simulink model "huxley_sim"  (R2021b)
settings: Solver=VariableStepAuto  StartTime=0.0  StopTime=2  RelTol=1e-3
values from neighbouring files (symbols this model uses):
  gK = 36    [huxley.m]
  gL = 0.3    [huxley.m]
  gNa = 120    [huxley.m]
  VK = -77    [huxley.m]
  VL = -54.4    [huxley.m]
  VNa = 50    [huxley.m]
  Vrest = -60    [huxley.m]
settings Model: Creator=eraym  LastModifiedBy=eraym

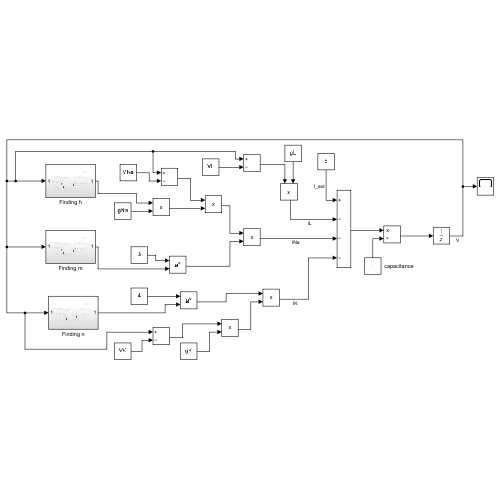
[thumbnail: Simulink's stored preview of the top-level diagram]
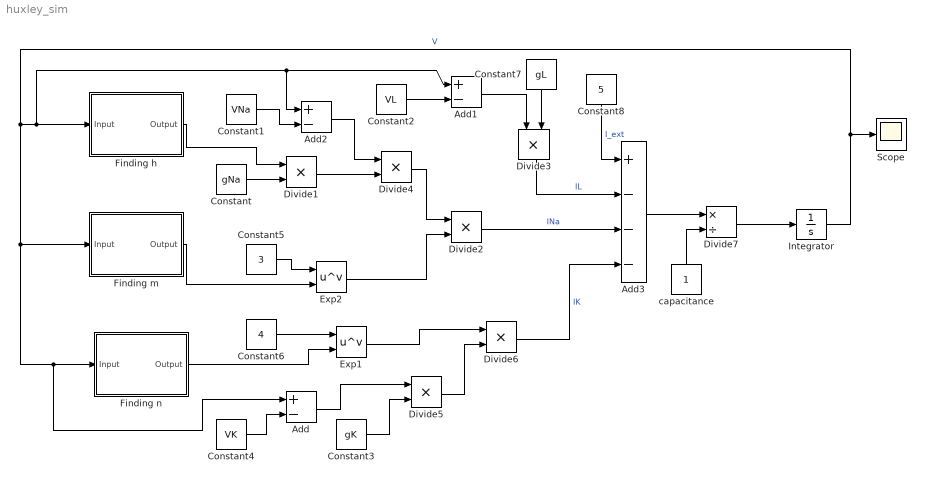
== system huxley_sim ==
  Add : Sum  Inputs=+-
  Add1 : Sum  Inputs=+-
  Add2 : Sum  Inputs=+-
  Add3 : Sum  Inputs=+---
  Constant : Constant  Value=gNa
  Constant1 : Constant  Value=VNa
  Constant2 : Constant  Value=VL
  Constant3 : Constant  Value=gK
  Constant4 : Constant  Value=VK
  Constant5 : Constant  Value=3
  Constant6 : Constant  Value=4
  Constant7 : Constant  Value=gL
  Constant8 : Constant  Value=5
  Divide{1..6} (6 alike) : Product  Inputs=**
  Divide7 : Product  Inputs=*/
  Exp1 : Math  Operator=pow  SaturateOnIntegerOverflow=on
  Exp2 : Math  Operator=pow  SaturateOnIntegerOverflow=on
  Finding h : Subsystem
  Finding m : Subsystem
  Finding n : Subsystem
  Integrator : Integrator
  Scope : Scope
  capacitance : Constant
  wires:
  Finding h/1(Output) -> Divide1/1
  Constant/1 -> Divide1/2
  Divide1/1 -> Divide4/2
  Add2/1 -> Divide4/1
  Constant1/1 -> Add2/2
  Divide4/1 -> Divide2/1
  Finding m/1(Output) -> Exp2/2
  Constant5/1 -> Exp2/1
  Exp2/1 -> Divide2/2
  Divide2/1 -> Add3/3  "INa"
  Divide6/1 -> Add3/4  "IK"
  Finding n/1(Output) -> Exp1/2
  Constant6/1 -> Exp1/1
  Exp1/1 -> Divide6/1
  Divide5/1 -> Divide6/2
  Constant3/1 -> Divide5/2
  Add/1 -> Divide5/1
  Constant4/1 -> Add/2
  Add3/1 -> Divide7/1
  capacitance/1 -> Divide7/2
  Divide7/1 -> Integrator/1
  Integrator/1 -> Scope/1, Add2/1, Add1/1, Finding h/1(Input), Add/1, Finding n/1(Input), Finding m/1(Input)  "V"
  Constant2/1 -> Add1/2
  Add1/1 -> Divide3/1
  Divide3/1 -> Add3/2  "IL"
  Constant7/1 -> Divide3/2
  Constant8/1 -> Add3/1  "I_ext"

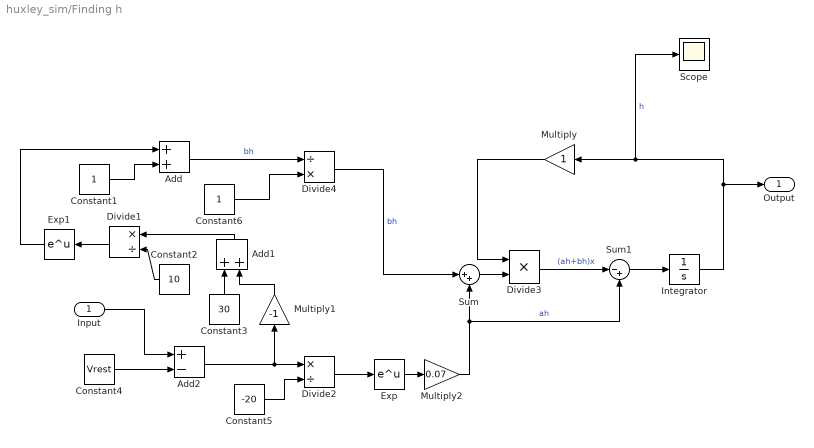
== system huxley_sim/Finding h ==
  Input : Inport
  Add : Sum
  Add1 : Sum
  Add2 : Sum  Inputs=+-
  Constant1 : Constant
  Constant2 : Constant  Value=10
  Constant3 : Constant  Value=30
  Constant4 : Constant  Value=Vrest
  Constant5 : Constant  Value=-20
  Constant6 : Constant
  Divide1 : Product  Inputs=*/
  Divide2 : Product  Inputs=*/
  Divide3 : Product  Inputs=**
  Divide4 : Product  Inputs=/*
  Exp : Math  SaturateOnIntegerOverflow=on
  Exp1 : Math  SaturateOnIntegerOverflow=on
  Integrator : Integrator
  Multiply : Gain
  Multiply1 : Gain  Gain=-1
  Multiply2 : Gain  Gain=0.07
  Scope : Scope
  Sum : Sum  Inputs=|++
  Sum1 : Sum  Inputs=|-+
  Output : Outport
  wires:
  Constant5/1 -> Divide2/2
  Input/1 -> Add2/1
  Sum/1 -> Divide3/2
  Add2/1 -> Divide2/1, Multiply1/1
  Divide1/1 -> Exp1/1
  Constant2/1 -> Divide1/2
  Divide2/1 -> Exp/1
  Exp/1 -> Multiply2/1
  Constant3/1 -> Add1/1
  Constant1/1 -> Add/2
  Add1/1 -> Divide1/1
  Exp1/1 -> Add/1
  Integrator/1 -> Output/1, Multiply/1, Scope/1  "h"
  Constant4/1 -> Add2/2
  Multiply1/1 -> Add1/2
  Multiply2/1 -> Sum1/2, Sum/2  "ah"
  Multiply/1 -> Divide3/1
  Divide4/1 -> Sum/1  "bh"
  Divide3/1 -> Sum1/1  "(ah+bh)x"
  Sum1/1 -> Integrator/1
  Add/1 -> Divide4/1  "bh"
  Constant6/1 -> Divide4/2

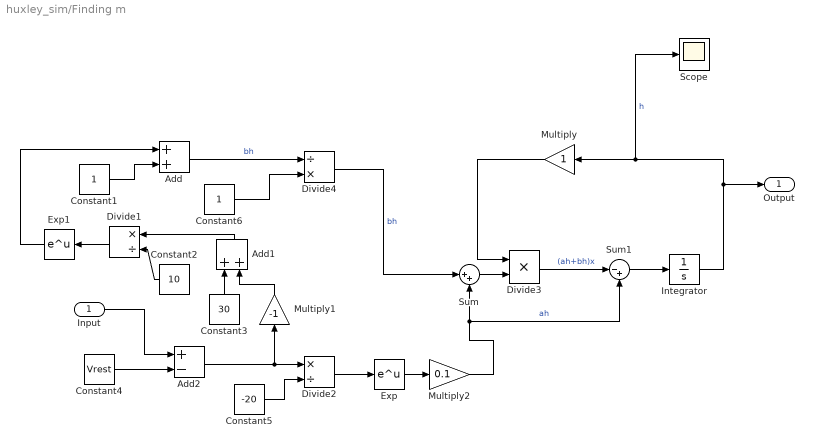
== system huxley_sim/Finding m ==
  Input : Inport
  Add : Sum
  Add1 : Sum
  Add2 : Sum  Inputs=+-
  Constant1 : Constant
  Constant2 : Constant  Value=10
  Constant3 : Constant  Value=30
  Constant4 : Constant  Value=Vrest
  Constant5 : Constant  Value=-20
  Constant6 : Constant
  Divide1 : Product  Inputs=*/
  Divide2 : Product  Inputs=*/
  Divide3 : Product  Inputs=**
  Divide4 : Product  Inputs=/*
  Exp : Math  SaturateOnIntegerOverflow=on
  Exp1 : Math  SaturateOnIntegerOverflow=on
  Integrator : Integrator
  Multiply : Gain
  Multiply1 : Gain  Gain=-1
  Multiply2 : Gain  Gain=0.1
  Scope : Scope
  Sum : Sum  Inputs=|++
  Sum1 : Sum  Inputs=|-+
  Output : Outport
  wires:
  Constant5/1 -> Divide2/2
  Input/1 -> Add2/1
  Sum/1 -> Divide3/2
  Add2/1 -> Divide2/1, Multiply1/1
  Divide1/1 -> Exp1/1
  Constant2/1 -> Divide1/2
  Divide2/1 -> Exp/1
  Exp/1 -> Multiply2/1
  Constant3/1 -> Add1/1
  Constant1/1 -> Add/2
  Add1/1 -> Divide1/1
  Exp1/1 -> Add/1
  Integrator/1 -> Output/1, Multiply/1, Scope/1  "h"
  Constant4/1 -> Add2/2
  Multiply1/1 -> Add1/2
  Multiply2/1 -> Sum1/2, Sum/2  "ah"
  Multiply/1 -> Divide3/1
  Divide4/1 -> Sum/1  "bh"
  Divide3/1 -> Sum1/1  "(ah+bh)x"
  Sum1/1 -> Integrator/1
  Add/1 -> Divide4/1  "bh"
  Constant6/1 -> Divide4/2

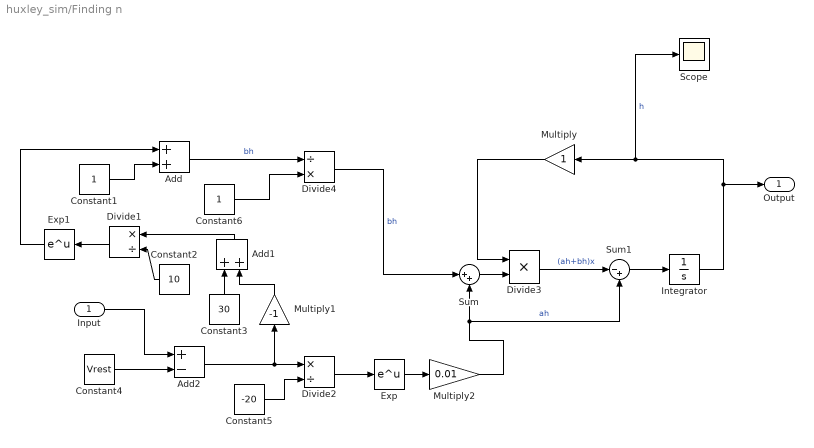
== system huxley_sim/Finding n ==
  Input : Inport
  Add : Sum
  Add1 : Sum
  Add2 : Sum  Inputs=+-
  Constant1 : Constant
  Constant2 : Constant  Value=10
  Constant3 : Constant  Value=30
  Constant4 : Constant  Value=Vrest
  Constant5 : Constant  Value=-20
  Constant6 : Constant
  Divide1 : Product  Inputs=*/
  Divide2 : Product  Inputs=*/
  Divide3 : Product  Inputs=**
  Divide4 : Product  Inputs=/*
  Exp : Math  SaturateOnIntegerOverflow=on
  Exp1 : Math  SaturateOnIntegerOverflow=on
  Integrator : Integrator
  Multiply : Gain
  Multiply1 : Gain  Gain=-1
  Multiply2 : Gain  Gain=0.01
  Scope : Scope
  Sum : Sum  Inputs=|++
  Sum1 : Sum  Inputs=|-+
  Output : Outport
  wires:
  Constant5/1 -> Divide2/2
  Input/1 -> Add2/1
  Sum/1 -> Divide3/2
  Add2/1 -> Divide2/1, Multiply1/1
  Divide1/1 -> Exp1/1
  Constant2/1 -> Divide1/2
  Divide2/1 -> Exp/1
  Exp/1 -> Multiply2/1
  Constant3/1 -> Add1/1
  Constant1/1 -> Add/2
  Add1/1 -> Divide1/1
  Exp1/1 -> Add/1
  Integrator/1 -> Output/1, Multiply/1, Scope/1  "h"
  Constant4/1 -> Add2/2
  Multiply1/1 -> Add1/2
  Multiply2/1 -> Sum1/2, Sum/2  "ah"
  Multiply/1 -> Divide3/1
  Divide4/1 -> Sum/1  "bh"
  Divide3/1 -> Sum1/1  "(ah+bh)x"
  Sum1/1 -> Integrator/1
  Add/1 -> Divide4/1  "bh"
  Constant6/1 -> Divide4/2
